simulink model "Monorail_Auxiliary_Power_Unit"  (R2021b)
settings: Solver=ode1  StartTime=0.0  StopTime=2.00  FixedStep=1e-06  MaxStep=1e-4  RelTol=1e-3
InitFcn:
  | %Input
  | V_supply_max = 910;
  | V_supply_min = 490;
  | V_supply_nom = 750;
  | R_supply = 1e-06;
  | L_in = 0.5e-03;
  | C_in = 215e-06;
  | R_Precharge = 1;
  | 
  | %PSFB_Voltage_Control
  | t_psfb_on = 0.05;
  | f_sw = 10e03;
  | V_dc_ref = 700;
  | V_dc_init = 450;
  | V_bat_ref = 24;
  | V_bat_init = 14;
  | Count_prd = 5000;
  | Half_prd = 2500;
  | Half_prd_fix = 2700;
  | Half_prd_var = 2300;
  | t_softstart = 100e-03;
  | Scale_factor_High = 1/737;
  | Scale_factor_Low = 1/48;
  | Kp_psfb = 2;
  | Ki_psfb =20;
  | Kp_feed = 0.00001;
  | PI_max = 1;
  | PI_min = 0;
  | t_enable = 1e-03;
  | Dead_prd = 1e-03
  | 
  | %PSFB_Current_Control
  | Scale_factor_i = 1/800;
  | I_cnst = 450;
  | I_over = 460;
  | Kp_psfb_i = 10;
  | Ki_psfb_i = 20;
  | 
  | %HF_Transformer
  | P_txf = 50e03;
  | f_txf = 10e03;
  | V_pri_txf = 1e03;
  | V_sec_high_txf = 720;
  | V_sec_low_txf = 27;
  | 
  | %DC_Link
  | L_filt = 1e-03;
  | C_filt = 215e-06;
  | R_Bleeder_700V = 0.5e03;
  | R_Bleeder_24V = 1e03
  | 
  | %Inverter_Control
  | t_inv_on = 1.5;
  | f_fund = 50;
  | V_phase_ref = 240;
  | Scale_factor_inv = 1/50e03;
  | Kp_inv = 0.05;
  | Ki_inv = 0.1;
  | PI_inv_max = 1;
  | PI_inv_min = -1;
  | ... (+27 lines)
undefined symbols (not defined in the file): Ion, Lithium
libraries: spsSeriesRLCBranchLib x35, spsIGBTDiodeLib x14, spsDiodeLib x13, spsMeanLib x11, spsBreakerLib x9, spsVoltageMeasurementLib x9, simulink x8, spsRMSLib x8, spsCurrentMeasurementLib x6, dspfdesign x6, spsabctodq0Lib x4, spsLinearTransformerLib x2
(part 2 of 3)

== system Monorail_Auxiliary_Power_Unit/First Stage/PSFB Pulse Generator/Loop Select ==
  Fixed Pulses Voltage Loop : Inport
  Variable Pulses Volatge Loop : Inport  Port=2
  OverCurrent Status : Inport  Port=3
  Fixed Pulses Current Loop : Inport  Port=4
  Variable Pulses Current Loop : Inport  Port=5
  Switch : Switch  Criteria=u2 > Threshold
  Switch1 : Switch  Criteria=u2 > Threshold
  Fixed Pulses : Outport
  Variable Pulses : Outport  Port=2
  wires:
  Switch/1 -> Fixed Pulses/1
  OverCurrent Status/1 -> Switch/2, Switch1/2
  Variable Pulses Current Loop/1 -> Switch1/3
  Variable Pulses Volatge Loop/1 -> Switch1/1
  Fixed Pulses Voltage Loop/1 -> Switch/1
  Switch1/1 -> Variable Pulses/1
  Fixed Pulses Current Loop/1 -> Switch/3

== system Monorail_Auxiliary_Power_Unit/First Stage/PSFB Pulse Generator/Voltage Loop ==
  Vi : Inport
  Vo 700V : Inport  Port=2
  Vo 24V : Inport  Port=3
  Fbk Sel : Inport  Port=4
  Carrier Wave Generator : Subsystem
  Close Loop : Subsystem
  Comparator : Subsystem
  Modulating Wave Generator : Subsystem
  Pulses for Fixed PSFB : Subsystem
  Pulses for Variable PSFB : Subsystem
  Fixed Pulses : Outport
  Variable Pulses : Outport  Port=2
  wires:
  Pulses for Fixed PSFB/1(Fixed Pulses) -> Fixed Pulses/1
  Comparator/1(Fixed PSFB R Top Pulse) -> Pulses for Fixed PSFB/1(Fixed PSFB R Top Pulse)
  Carrier Wave Generator/1(Carrier Wave) -> Comparator/1(Carrier Wave)
  Fbk Sel/1 -> Close Loop/4(Fbk Sel)
  Close Loop/1(Phase Shift) -> Pulses for Variable PSFB/2(Phase Shift)
  Modulating Wave Generator/2(Variable Modulating Wave) -> Comparator/3(Variable Modulating Wave)
  Vo 24V/1 -> Close Loop/3(Vdc 24V)
  Modulating Wave Generator/1(Fixed Modulating Wave) -> Comparator/2(Fixed Modulating Wave)
  Vo 700V/1 -> Close Loop/2(Vdc 700V)
  Comparator/2(Variable PSFB R Top Pulse) -> Pulses for Variable PSFB/1(Variable PSFB R Top Pulse)
  Pulses for Variable PSFB/1(Variable Pulses) -> Variable Pulses/1
  Vi/1 -> Close Loop/1(Vi)

== system Monorail_Auxiliary_Power_Unit/Second Stage/Pulse Generator/Current Loop ==
  I fbk : Inport
  I Feedback : Subsystem
  I Modulation Index : Display
  I PI Block : Subsystem
  I Reference : Subsystem
  Overcurrent Status Check : Subsystem
  I PI Out : Outport
  I Theta : Outport  Port=2
  Inverter Overcurrent Status : Outport  Port=3
  wires:
  I PI Block/1(I PI Out) -> I PI Out/1
  I Feedback/1(I dq0) -> I PI Block/2(I Feedback)
  I fbk/1 -> I Feedback/1(I fbk), Overcurrent Status Check/1(I fbk)
  I Reference/2(I ThetaIdeal) -> [ITheta]
  [ITheta] -> I Feedback/2(I Theta), I Theta/1
  I Reference/1(I dq0) -> I PI Block/1(I Reference)
  I PI Block/2(I Modulation Index) -> I Modulation Index/1
  Overcurrent Status Check/1(Inverter Overcurrent Status) -> Inverter Overcurrent Status/1

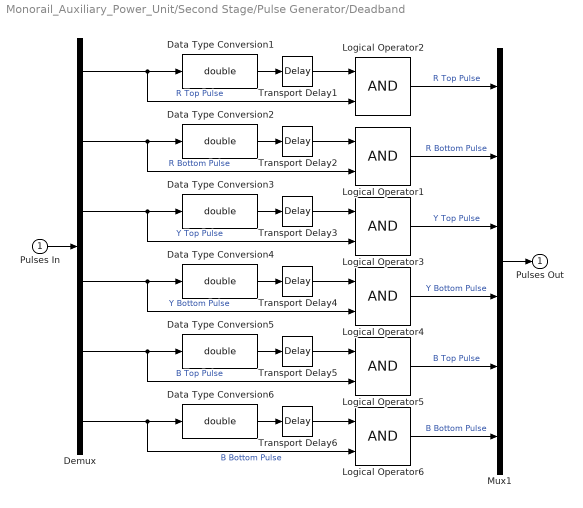
== system Monorail_Auxiliary_Power_Unit/Second Stage/Pulse Generator/Deadband ==
  Pulses In : Inport
  Data Type Conversion{1..6} (6 alike) : DataTypeConversion  OutDataTypeStr=double
  Demux : Demux  Outputs=6
  Logical Operator{1..6} (6 alike) : Logic  IconShape=distinctive  AllPortsSameDT=off  OutDataTypeStr=boolean
  Mux1 : Mux  Inputs=6
  Transport Delay{1..6} (6 alike) : TransportDelay  DelayTime=t_dead
  Pulses Out : Outport
  wires:
  Transport Delay2/1 -> Logical Operator1/1
  Data Type Conversion4/1 -> Transport Delay4/1
  Transport Delay3/1 -> Logical Operator3/1
  Transport Delay5/1 -> Logical Operator5/1
  Demux/2 -> Logical Operator1/2, Data Type Conversion2/1  "R Bottom Pulse"
  Data Type Conversion1/1 -> Transport Delay1/1
  Demux/1 -> Logical Operator2/2, Data Type Conversion1/1  "R Top Pulse"
  Transport Delay1/1 -> Logical Operator2/1
  Demux/4 -> Logical Operator4/2, Data Type Conversion4/1  "Y Bottom Pulse"
  Data Type Conversion3/1 -> Transport Delay3/1
  Transport Delay4/1 -> Logical Operator4/1
  Demux/3 -> Logical Operator3/2, Data Type Conversion3/1  "Y Top Pulse"
  Data Type Conversion2/1 -> Transport Delay2/1
  Data Type Conversion5/1 -> Transport Delay5/1
  Demux/5 -> Logical Operator5/2, Data Type Conversion5/1  "B Top Pulse"
  Demux/6 -> Logical Operator6/2, Data Type Conversion6/1  "B Bottom Pulse"
  Transport Delay6/1 -> Logical Operator6/1
  Data Type Conversion6/1 -> Transport Delay6/1
  Mux1/1 -> Pulses Out/1
  Logical Operator3/1 -> Mux1/3  "Y Top Pulse"
  Logical Operator2/1 -> Mux1/1  "R Top Pulse"
  Logical Operator5/1 -> Mux1/5  "B Top Pulse"
  Logical Operator1/1 -> Mux1/2  "R Bottom Pulse"
  Logical Operator4/1 -> Mux1/4  "Y Bottom Pulse"
  Logical Operator6/1 -> Mux1/6  "B Bottom Pulse"
  Pulses In/1 -> Demux/1

== system Monorail_Auxiliary_Power_Unit/Second Stage/Pulse Generator/Loop Select ==
  I PI : Inport
  I Theta : Inport  Port=2
  Inverter Overcurrent Status : Inport  Port=3
  V PI : Inport  Port=4
  V Theta : Inport  Port=5
  DQ0 Switch : Switch  Criteria=u2 > Threshold  Threshold=1/2
  Theta Switch : Switch  Criteria=u2 > Threshold  Threshold=1/2
  DQ0 : Outport
  Theta : Outport  Port=2
  wires:
  V Theta/1 -> Theta Switch/3
  Inverter Overcurrent Status/1 -> DQ0 Switch/2, Theta Switch/2
  I PI/1 -> DQ0 Switch/1
  V PI/1 -> DQ0 Switch/3
  DQ0 Switch/1 -> DQ0/1
  Theta Switch/1 -> Theta/1
  I Theta/1 -> Theta Switch/1

== system Monorail_Auxiliary_Power_Unit/Second Stage/Pulse Generator/Pulse ==
  dq0 : Inport
  Theta : Inport  Port=2
  Gate Pulses : Subsystem
  IPARK_MACRO : Subsystem
  SVGEN_DQ : Subsystem
  Pulses : Outport
  wires:
  SVGEN_DQ/1(SW) -> Gate Pulses/1(SW)
  Gate Pulses/1(Pulses) -> Pulses/1
  IPARK_MACRO/1(Alpha) -> SVGEN_DQ/1(Alpha)
  IPARK_MACRO/2(Beta) -> SVGEN_DQ/2(Beta)
  dq0/1 -> IPARK_MACRO/1(DQ0)
  Theta/1 -> IPARK_MACRO/2(Theta)

== system Monorail_Auxiliary_Power_Unit/Second Stage/Pulse Generator/Voltage Loop ==
  V fbk : Inport
  V Feedback : Subsystem
  V Modulation Index : Display
  V PI Block : Subsystem
  V Reference : Subsystem
  V PI Out : Outport
  V Theta : Outport  Port=2
  wires:
  V PI Block/2(V Modulation Index) -> V Modulation Index/1
  V Reference/1(V dq0) -> V PI Block/1(V Reference)
  [VTheta] -> V Theta/1, V Feedback/2(Theta)
  V Reference/2(V ThetaIdeal) -> [VTheta]
  V fbk/1 -> V Feedback/1(fbk)
  V Feedback/1(dq0) -> V PI Block/2(V Feedback)
  V PI Block/1(V PI Out) -> V PI Out/1

== system Monorail_Auxiliary_Power_Unit/First Stage/PSFB Pulse Generator/Current Loop/Carrier Wave Generator ==
  Repeating Sequence : simulink/Sources/Repeating Sequence  rep_seq_t=[0 (1/f_sw)/2 1/f_sw]  rep_seq_y=[0 Count_prd 0]
  Saturation5 : Saturate  UpperLimit=Count_prd  LowerLimit=0
  Carrier Wave : Outport
  wires:
  Saturation5/1 -> Carrier Wave/1  "Limited Carrier Wave"
  Repeating Sequence/1 -> Saturation5/1  "Carrier Wave"

== system Monorail_Auxiliary_Power_Unit/First Stage/PSFB Pulse Generator/Current Loop/Close Loop ==
  Ibat : Inport
  Error Signal Generator : Subsystem
  OverCurrent Fault Check : Subsystem
  PI Controller : Subsystem
  Duty : Outport
  OverCurrent Status : Outport  Port=2
  wires:
  Ibat/1 -> OverCurrent Fault Check/1(I bat), Error Signal Generator/1(Ibat)
  OverCurrent Fault Check/1(OverCurrent Status) -> OverCurrent Status/1
  PI Controller/1(Duty) -> Duty/1
  Error Signal Generator/1(Error Signal) -> PI Controller/1(Error Signal)

== system Monorail_Auxiliary_Power_Unit/First Stage/PSFB Pulse Generator/Current Loop/Comparator ==
  Carrier Wave : Inport
  Fixed Modulating Wave : Inport  Port=2
  Variable Modulating Wave : Inport  Port=3
  Relational Operator2 : RelationalOperator  OutDataTypeStr=boolean  RndMeth=Nearest
  Relational Operator3 : RelationalOperator  Operator=<=  OutDataTypeStr=boolean  RndMeth=Nearest
  Fixed PSFB R Top Pulse : Outport
  Variable PSFB R Top Pulse : Outport  Port=2
  wires:
  Variable Modulating Wave/1 -> Relational Operator3/2
  Relational Operator3/1 -> Variable PSFB R Top Pulse/1  "Pulse"
  Relational Operator2/1 -> Fixed PSFB R Top Pulse/1  "Pulse"
  Carrier Wave/1 -> Relational Operator2/1, Relational Operator3/1
  Fixed Modulating Wave/1 -> Relational Operator2/2

== system Monorail_Auxiliary_Power_Unit/First Stage/PSFB Pulse Generator/Current Loop/Modulating Wave Generator ==
  Duty : Inport
  Constant2 : Constant  Value=Half_prd_fix
  Constant3 : Constant  Value=Half_prd_var
  Saturation : Saturate  UpperLimit=Half_prd_var  LowerLimit=0
  Saturation1 : Saturate  UpperLimit=Count_prd  LowerLimit=Half_prd_fix
  Sum3 : Sum  Inputs=|+-
  Sum4 : Sum  Inputs=|++
  Fixed Modulating Wave : Outport
  Variable Modulating Wave : Outport  Port=2
  wires:
  Duty/1 -> Sum4/2, Sum3/2
  Constant2/1 -> Sum4/1
  Constant3/1 -> Sum3/1
  Sum4/1 -> Saturation1/1
  Sum3/1 -> Saturation/1
  Saturation/1 -> Variable Modulating Wave/1
  Saturation1/1 -> Fixed Modulating Wave/1

== system Monorail_Auxiliary_Power_Unit/First Stage/PSFB Pulse Generator/Current Loop/Pulses for Fixed PSFB ==
  Fixed PSFB R Top Pulse : Inport
  Data Type Conversion1 : DataTypeConversion  OutDataTypeStr=boolean
  Data Type Conversion6 : DataTypeConversion  OutDataTypeStr=double
  Mux : Mux  Inputs=2
  Rate Transition : RateTransition  Commented=through
  Transport Delay1 : TransportDelay  DelayTime=(180/360)*(1/f_sw)
  Fixed Pulses : Outport
  wires:
  Fixed PSFB R Top Pulse/1 -> Mux/1, Data Type Conversion6/1  "Fixed PSFB R Top Pulse"
  Data Type Conversion1/1 -> Mux/2  "Fixed PSFB Y Top Pulse"
  Rate Transition/1 -> Fixed Pulses/1
  Mux/1 -> Rate Transition/1
  Transport Delay1/1 -> Data Type Conversion1/1
  Data Type Conversion6/1 -> Transport Delay1/1

== system Monorail_Auxiliary_Power_Unit/First Stage/PSFB Pulse Generator/Current Loop/Pulses for Variable PSFB ==
  Fixed PSFB R Top Pulse : Inport
  Data Type Conversion1 : DataTypeConversion  OutDataTypeStr=boolean
  Data Type Conversion6 : DataTypeConversion  OutDataTypeStr=double
  Mux : Mux  Inputs=2
  Rate Transition : RateTransition  Commented=through
  Transport Delay1 : TransportDelay  DelayTime=(180/360)*(1/f_sw)
  Fixed Pulses : Outport
  wires:
  Data Type Conversion6/1 -> Transport Delay1/1
  Transport Delay1/1 -> Data Type Conversion1/1
  Mux/1 -> Rate Transition/1
  Rate Transition/1 -> Fixed Pulses/1
  Data Type Conversion1/1 -> Mux/2  "Fixed PSFB Y Top Pulse"
  Fixed PSFB R Top Pulse/1 -> Data Type Conversion6/1, Mux/1  "Fixed PSFB R Top Pulse"

== system Monorail_Auxiliary_Power_Unit/First Stage/PSFB Pulse Generator/Voltage Loop/Carrier Wave Generator ==
  Repeating Sequence : simulink/Sources/Repeating Sequence  rep_seq_t=[0 (1/f_sw)/2 1/f_sw]  rep_seq_y=[0 Count_prd 0]
  Saturation5 : Saturate  UpperLimit=Count_prd  LowerLimit=0
  Carrier Wave : Outport
  wires:
  Repeating Sequence/1 -> Saturation5/1  "Carrier Wave"
  Saturation5/1 -> Carrier Wave/1  "Limited Carrier Wave"

== system Monorail_Auxiliary_Power_Unit/First Stage/PSFB Pulse Generator/Voltage Loop/Close Loop ==
  Vi : Inport
  Vdc 700V : Inport  Port=2
  Vdc 24V : Inport  Port=3
  Fbk Sel : Inport  Port=4
  Feedback : Subsystem
  Feedforward : Subsystem
  Gain6 : Gain  Gain=(180/360)*(1/f_sw)
  Sum : Sum  Inputs=|++
  Phase Shift : Outport
  wires:
  Vdc 700V/1 -> Feedback/1(Vdc 700V)
  Vdc 24V/1 -> Feedback/2(Vdc 24V)
  Fbk Sel/1 -> Feedback/3(Fbk Sel)
  Feedback/1(PI Out) -> Sum/2
  Sum/1 -> Gain6/1
  Gain6/1 -> Phase Shift/1
  Vi/1 -> Feedforward/1(V supply)
  Feedforward/1(P Out) -> Sum/1

== system Monorail_Auxiliary_Power_Unit/First Stage/PSFB Pulse Generator/Voltage Loop/Comparator ==
  Carrier Wave : Inport
  Fixed Modulating Wave : Inport  Port=2
  Variable Modulating Wave : Inport  Port=3
  Relational Operator2 : RelationalOperator  OutDataTypeStr=boolean  RndMeth=Nearest
  Relational Operator3 : RelationalOperator  Operator=<=  OutDataTypeStr=boolean  RndMeth=Nearest
  Fixed PSFB R Top Pulse : Outport
  Variable PSFB R Top Pulse : Outport  Port=2
  wires:
  Fixed Modulating Wave/1 -> Relational Operator2/2
  Carrier Wave/1 -> Relational Operator3/1, Relational Operator2/1
  Relational Operator2/1 -> Fixed PSFB R Top Pulse/1  "Pulse"
  Relational Operator3/1 -> Variable PSFB R Top Pulse/1  "Pulse"
  Variable Modulating Wave/1 -> Relational Operator3/2

== system Monorail_Auxiliary_Power_Unit/First Stage/PSFB Pulse Generator/Voltage Loop/Modulating Wave Generator ==
  Constant1 : Constant  Value=Count_prd
  Ramp2 : simulink/Sources/Ramp  slope=((Count_prd/2)-Dead_prd)/t_softstart  start=0  InitialOutput=0
  Saturation : Saturate  UpperLimit=Half_prd_var  LowerLimit=0
  Saturation4 : Saturate  UpperLimit=Count_prd  LowerLimit=Half_prd_fix
  Saturation6 : Saturate  UpperLimit=Half_prd_var  LowerLimit=0
  Sum2 : Sum  Inputs=|+-
  Fixed Modulating Wave : Outport
  Variable Modulating Wave : Outport  Port=2
  wires:
  Saturation/1 -> Sum2/2, Saturation6/1  "Actual Modulating Wave"
  Sum2/1 -> Saturation4/1  "Actual Modulating Wave"
  Saturation4/1 -> Fixed Modulating Wave/1  "Saturated Modulating Wave"
  Constant1/1 -> Sum2/1  "TBPRD"
  Ramp2/1 -> Saturation/1  "Initial Modulating Wave"
  Saturation6/1 -> Variable Modulating Wave/1  "Saturated Modulating Wave"

== system Monorail_Auxiliary_Power_Unit/First Stage/PSFB Pulse Generator/Voltage Loop/Pulses for Fixed PSFB ==
  Fixed PSFB R Top Pulse : Inport
  Data Type Conversion1 : DataTypeConversion  OutDataTypeStr=boolean
  Data Type Conversion6 : DataTypeConversion  OutDataTypeStr=double
  Mux : Mux  Inputs=2
  Rate Transition : RateTransition
  Transport Delay1 : TransportDelay  DelayTime=(180/360)*(1/f_sw)
  Fixed Pulses : Outport
  wires:
  Data Type Conversion6/1 -> Transport Delay1/1
  Transport Delay1/1 -> Data Type Conversion1/1
  Mux/1 -> Rate Transition/1
  Rate Transition/1 -> Fixed Pulses/1
  Data Type Conversion1/1 -> Mux/2  "Fixed PSFB Y Top Pulse"
  Fixed PSFB R Top Pulse/1 -> Data Type Conversion6/1, Mux/1  "Fixed PSFB R Top Pulse"

== system Monorail_Auxiliary_Power_Unit/First Stage/PSFB Pulse Generator/Voltage Loop/Pulses for Variable PSFB ==
  Variable PSFB R Top Pulse : Inport
  Phase Shift : Inport  Port=2
  Data Type Conversion2 : DataTypeConversion  OutDataTypeStr=double
  Data Type Conversion3 : DataTypeConversion  OutDataTypeStr=boolean
  Data Type Conversion5 : DataTypeConversion  OutDataTypeStr=boolean
  Mux1 : Mux  Inputs=2
  Rate Transition1 : RateTransition
  Transport Delay2 : TransportDelay  DelayTime=(180/360)*(1/f_sw)
  Variable Transport Delay : VariableTransportDelay  MaximumDelay=1/f_sw
  Variable Pulses : Outport
  wires:
  Phase Shift/1 -> Variable Transport Delay/2
  Data Type Conversion5/1 -> Mux1/1  "Variable PSFB R Top Pulse"
  Mux1/1 -> Rate Transition1/1
  Transport Delay2/1 -> Data Type Conversion3/1
  Variable PSFB R Top Pulse/1 -> Data Type Conversion2/1
  Data Type Conversion3/1 -> Mux1/2  "Variable PSFB Y Top Pulse"
  Data Type Conversion2/1 -> Variable Transport Delay/1
  Variable Transport Delay/1 -> Data Type Conversion5/1, Transport Delay2/1
  Rate Transition1/1 -> Variable Pulses/1

== system Monorail_Auxiliary_Power_Unit/Second Stage/Pulse Generator/Current Loop/I Feedback ==
  I fbk : Inport
  I Theta : Inport  Port=2
  Demux : Demux  Outputs=3
  Gain5 : Gain  Gain=Scale_factor_Iinv
  Lowpass Filter BR : dspfdesign/Lowpass Filter  Commented=through  FilterType=FIR  DesignForMinimumOrder=on  FilterOrder=50  PassbandFrequency=50  StopbandFrequency=1e03  PassbandRipple=0.1  StopbandAttenuation=100  InheritSampleRate=off  SampleRate=44100  SimulateUsing=Interpreted execution  roundingMode=Floor  coeffsDataTypeStr=fixdt(1,16)
  Lowpass Filter RY : dspfdesign/Lowpass Filter  Commented=through  FilterType=FIR  DesignForMinimumOrder=on  FilterOrder=50  PassbandFrequency=50  StopbandFrequency=1e03  PassbandRipple=0.1  StopbandAttenuation=100  InheritSampleRate=off  SampleRate=44100  SimulateUsing=Interpreted execution  roundingMode=Floor  coeffsDataTypeStr=fixdt(1,16)
  Lowpass Filter YB : dspfdesign/Lowpass Filter  Commented=through  FilterType=FIR  DesignForMinimumOrder=on  FilterOrder=50  PassbandFrequency=50  StopbandFrequency=1e03  PassbandRipple=0.1  StopbandAttenuation=100  InheritSampleRate=off  SampleRate=44100  SimulateUsing=Interpreted execution  roundingMode=Floor  coeffsDataTypeStr=fixdt(1,16)
  Mux : Mux  Inputs=3
  abc to dq0 : spsabctodq0Lib/abc to dq0  Alignment=90 degrees behind phase A axis
  I dq0 : Outport
  wires:
  I fbk/1 -> Demux/1
  Demux/3 -> Lowpass Filter BR/1
  Demux/2 -> Lowpass Filter YB/1
  Demux/1 -> Lowpass Filter RY/1
  Lowpass Filter BR/1 -> Mux/3
  Lowpass Filter YB/1 -> Mux/2
  Lowpass Filter RY/1 -> Mux/1
  I Theta/1 -> abc to dq0/2
  Mux/1 -> Gain5/1
  abc to dq0/1 -> I dq0/1
  Gain5/1 -> abc to dq0/1

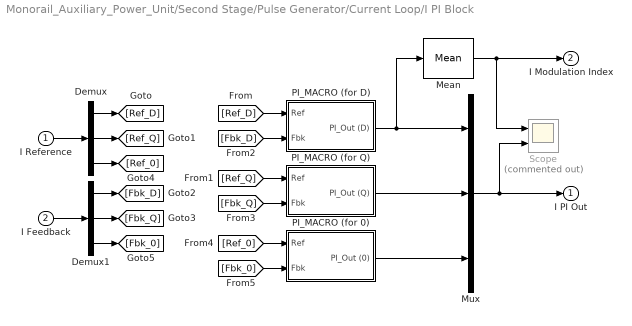
== system Monorail_Auxiliary_Power_Unit/Second Stage/Pulse Generator/Current Loop/I PI Block ==
  I Reference : Inport
  I Feedback : Inport  Port=2
  Demux : Demux  Outputs=3
  Demux1 : Demux  Outputs=3
  Mean : spsMeanLib/Mean  Freq=f_fund  Vinit=0  Ts=0
  Mux : Mux  Inputs=3
  PI_MACRO (for 0) : Subsystem
  PI_MACRO (for D) : Subsystem
  PI_MACRO (for Q) : Subsystem
  Scope : Scope  Commented=on  NumInputPorts=2
  I PI Out : Outport
  I Modulation Index : Outport  Port=2
  wires:
  PI_MACRO (for D)/1(PI_Out (D)) -> Mux/1, Mean/1
  Mean/1 -> I Modulation Index/1, Scope/1
  PI_MACRO (for 0)/1(PI_Out (0)) -> Mux/3
  [Ref_0] -> PI_MACRO (for 0)/1(Ref)
  [Fbk_0] -> PI_MACRO (for 0)/2(Fbk)
  I Reference/1 -> Demux/1
  I Feedback/1 -> Demux1/1
  [Fbk_Q] -> PI_MACRO (for Q)/2(Fbk)
  Demux1/2 -> [Fbk_Q]
  [Fbk_D] -> PI_MACRO (for D)/2(Fbk)
  Demux1/1 -> [Fbk_D]
  [Ref_Q] -> PI_MACRO (for Q)/1(Ref)
  Demux/2 -> [Ref_Q]
  [Ref_D] -> PI_MACRO (for D)/1(Ref)
  Demux/1 -> [Ref_D]
  Demux/3 -> [Ref_0]
  Demux1/3 -> [Fbk_0]
  PI_MACRO (for Q)/1(PI_Out (Q)) -> Mux/2
  Mux/1 -> Scope/2, I PI Out/1

== system Monorail_Auxiliary_Power_Unit/Second Stage/Pulse Generator/Current Loop/I Reference ==
  Constant : Constant  Value=2*pi/3
  Gain1 : Gain  Gain=I_Line_ref*sqrt(2)
  Gain2 : Gain  Gain=Scale_factor_Iinv
  Gain3 : Gain  Gain=I_Line_ref*sqrt(2)
  Gain4 : Gain  Gain=I_Line_ref*sqrt(2)
  I Theta : simulink/Sources/Repeating Sequence  rep_seq_t=[0 1/f_fund]  rep_seq_y=[0 2*pi]
  Mux2 : Mux  Inputs=3
  Sum1 : Sum  Inputs=|+-
  Sum2 : Sum  Inputs=|++
  Trigonometric Function : Trigonometry
  Trigonometric Function1 : Trigonometry
  Trigonometric Function2 : Trigonometry
  abc to dq0 : spsabctodq0Lib/abc to dq0  Alignment=90 degrees behind phase A axis
  I dq0 : Outport
  I ThetaIdeal : Outport  Port=2
  wires:
  [IThetaIdeal] -> I ThetaIdeal/1, abc to dq0/2
  Gain3/1 -> Mux2/2
  Gain1/1 -> Mux2/1
  Gain4/1 -> Mux2/3
  Gain2/1 -> abc to dq0/1
  I Theta/1 -> Sum2/1, Sum1/1, [IThetaIdeal], Trigonometric Function/1
  Mux2/1 -> Gain2/1
  abc to dq0/1 -> I dq0/1
  Constant/1 -> Sum1/2, Sum2/2
  Sum2/1 -> Trigonometric Function2/1
  Trigonometric Function/1 -> Gain1/1  "R"
  Trigonometric Function1/1 -> Gain3/1  "Y"
  Trigonometric Function2/1 -> Gain4/1  "B"
  Sum1/1 -> Trigonometric Function1/1

== system Monorail_Auxiliary_Power_Unit/Second Stage/Pulse Generator/Current Loop/Overcurrent Status Check ==
  I fbk : Inport
  Constant : Constant  Value=Iinvov
  Demux : Demux  Outputs=3
  GreaterThan1 : RelationalOperator  Operator=>  OutDataTypeStr=boolean  RndMeth=Simplest
  GreaterThan2 : RelationalOperator  Operator=>  OutDataTypeStr=boolean  RndMeth=Simplest
  GreaterThan3 : RelationalOperator  Operator=>  OutDataTypeStr=boolean  RndMeth=Simplest
  Logical Operator : Logic  Operator=OR  Inputs=3  IconShape=distinctive  AllPortsSameDT=off  OutDataTypeStr=boolean
  RMS1 : spsRMSLib/RMS  TrueRMS=on  Freq=f_fund  RMSInit=0  Ts=0
  RMS2 : spsRMSLib/RMS  TrueRMS=on  Freq=f_fund  RMSInit=0  Ts=0
  RMS3 : spsRMSLib/RMS  TrueRMS=on  Freq=f_fund  RMSInit=0  Ts=0
  Inverter Overcurrent Status : Outport
  wires:
  RMS1/1 -> GreaterThan1/1
  RMS2/1 -> GreaterThan2/1
  RMS3/1 -> GreaterThan3/1
  Constant/1 -> GreaterThan3/2, GreaterThan1/2, GreaterThan2/2
  GreaterThan1/1 -> Logical Operator/2
  Demux/1 -> RMS3/1
  GreaterThan2/1 -> Logical Operator/3
  Demux/2 -> RMS1/1
  Demux/3 -> RMS2/1
  GreaterThan3/1 -> Logical Operator/1
  Logical Operator/1 -> Inverter Overcurrent Status/1
  I fbk/1 -> Demux/1

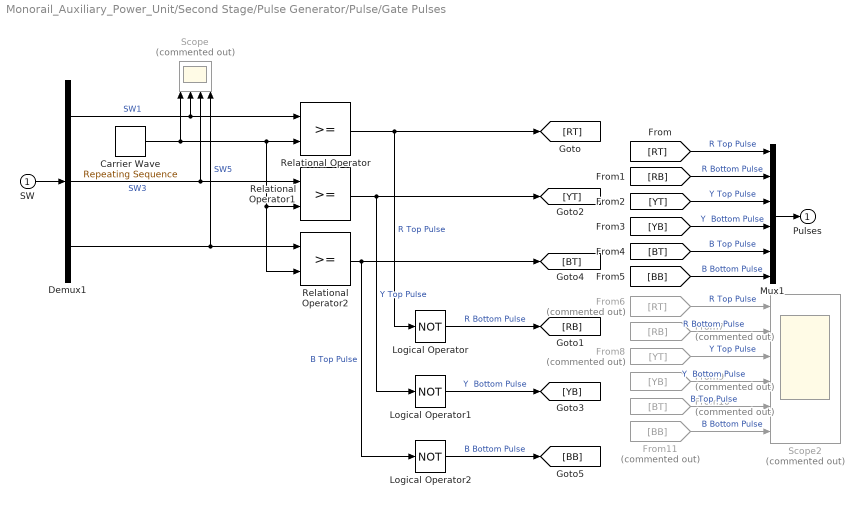
== system Monorail_Auxiliary_Power_Unit/Second Stage/Pulse Generator/Pulse/Gate Pulses ==
  SW : Inport
  Carrier Wave : simulink/Sources/Repeating Sequence  rep_seq_t=[0 (1/2e03)/2 1/2e03]  rep_seq_y=[0 1 0]
  Demux1 : Demux  Outputs=3
  From10 : From  Commented=on  GotoTag=BT
  From11 : From  Commented=on  GotoTag=BB
  From6 : From  Commented=on  GotoTag=RT
  From7 : From  Commented=on  GotoTag=RB
  From8 : From  Commented=on  GotoTag=YT
  From9 : From  Commented=on  GotoTag=YB
  Logical Operator : Logic  Operator=NOT  IconShape=distinctive  AllPortsSameDT=off  OutDataTypeStr=boolean
  Logical Operator1 : Logic  Operator=NOT  IconShape=distinctive  AllPortsSameDT=off  OutDataTypeStr=boolean
  Logical Operator2 : Logic  Operator=NOT  IconShape=distinctive  AllPortsSameDT=off  OutDataTypeStr=boolean
  Mux1 : Mux  Inputs=6
  Relational Operator : RelationalOperator  OutDataTypeStr=boolean  RndMeth=Nearest
  Relational Operator1 : RelationalOperator  OutDataTypeStr=boolean  RndMeth=Nearest
  Relational Operator2 : RelationalOperator  OutDataTypeStr=boolean  RndMeth=Nearest
  Scope : Scope  Commented=on  NumInputPorts=4
  Scope2 : Scope  Commented=on  NumInputPorts=6
  Pulses : Outport
  wires:
  Logical Operator/1 -> [RB]  "R Bottom Pulse"
  Logical Operator1/1 -> [YB]  "Y  Bottom Pulse"
  Demux1/2 -> Scope/3, Relational Operator1/1  "SW3"
  Demux1/3 -> Scope/4, Relational Operator2/1  "SW5"
  Logical Operator2/1 -> [BB]  "B Bottom Pulse"
  Demux1/1 -> Scope/2, Relational Operator/1  "SW1"
  Relational Operator2/1 -> [BT], Logical Operator2/1  "B Top Pulse"
  Relational Operator/1 -> Logical Operator/1, [RT]  "R Top Pulse"
  Carrier Wave/1 -> Relational Operator2/2, Relational Operator1/2, Relational Operator/2, Scope/1
  Relational Operator1/1 -> [YT], Logical Operator1/1  "Y Top Pulse"
  SW/1 -> Demux1/1
  Mux1/1 -> Pulses/1
  [YT] -> Mux1/3  "Y Top Pulse"
  [RT] -> Mux1/1  "R Top Pulse"
  [BT] -> Mux1/5  "B Top Pulse"
  [RB] -> Mux1/2  "R Bottom Pulse"
  [YB] -> Mux1/4  "Y  Bottom Pulse"
  [BB] -> Mux1/6  "B Bottom Pulse"
  From6/1 -> Scope2/1  "R Top Pulse"
  From7/1 -> Scope2/2  "R Bottom Pulse"
  From8/1 -> Scope2/3  "Y Top Pulse"
  From9/1 -> Scope2/4  "Y  Bottom Pulse"
  From10/1 -> Scope2/5  "B Top Pulse"
  From11/1 -> Scope2/6  "B Bottom Pulse"

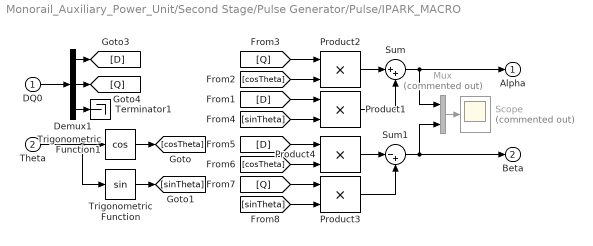
== system Monorail_Auxiliary_Power_Unit/Second Stage/Pulse Generator/Pulse/IPARK_MACRO ==
  DQ0 : Inport
  Theta : Inport  Port=2
  Demux1 : Demux  Outputs=3
  Mux : Mux  Commented=on  Inputs=2
  Product{1..4} (4 alike) : Product
  Scope : Scope  Commented=on
  Sum : Sum  Inputs=|++
  Sum1 : Sum  Inputs=|-+
  Terminator1 : Terminator
  Trigonometric Function : Trigonometry
  Trigonometric Function1 : Trigonometry  Operator=cos
  Alpha : Outport
  Beta : Outport  Port=2
  wires:
  Trigonometric Function1/1 -> [cosTheta]
  Trigonometric Function/1 -> [sinTheta]
  Theta/1 -> Trigonometric Function/1, Trigonometric Function1/1
  Demux1/3 -> Terminator1/1
  Demux1/1 -> [D]
  Demux1/2 -> [Q]
  Product2/1 -> Sum/1
  Product1/1 -> Sum/2
  Sum/1 -> Mux/1, Alpha/1
  Sum1/1 -> Beta/1, Mux/2
  Product3/1 -> Sum1/2
  Product4/1 -> Sum1/1
  [Q] -> Product2/1
  [cosTheta] -> Product2/2
  [D] -> Product1/1
  [sinTheta] -> Product1/2
  [D] -> Product4/1
  [cosTheta] -> Product4/2
  [Q] -> Product3/1
  [sinTheta] -> Product3/2
  DQ0/1 -> Demux1/1
  Mux/1 -> Scope/1

== system Monorail_Auxiliary_Power_Unit/Second Stage/Pulse Generator/Pulse/SVGEN_DQ ==
  Alpha : Inport
  Beta : Inport  Port=2
  Display : Display  Commented=on
  Scaling Block : Subsystem
  "Sector " : Scope  Commented=on
  Sector Determination : Subsystem
  Switching Time Calculation : Subsystem
  Temp calculation : Subsystem
  SW : Outport
  wires:
  Alpha/1 -> Temp calculation/1(Alpha)
  Sector Determination/1(Sector) -> Switching Time Calculation/2(Sector), "Sector "/1, Display/1
  Temp calculation/1(Temp) -> Switching Time Calculation/1(tmp), Sector Determination/1(Temp)
  Beta/1 -> Temp calculation/2(Beta)
  Switching Time Calculation/1(Switching Time) -> Scaling Block/1(In)
  Scaling Block/1(Out) -> SW/1

== system Monorail_Auxiliary_Power_Unit/Second Stage/Pulse Generator/Voltage Loop/V Feedback ==
  fbk : Inport
  Theta : Inport  Port=2
  Demux : Demux  Outputs=3
  Gain5 : Gain  Gain=Scale_factor_inv
  Lowpass Filter BR : dspfdesign/Lowpass Filter  Commented=through  FilterType=FIR  DesignForMinimumOrder=on  FilterOrder=50  PassbandFrequency=f_fund  StopbandFrequency=1e03  PassbandRipple=0.1  StopbandAttenuation=100  InheritSampleRate=off  SampleRate=44100  SimulateUsing=Interpreted execution  roundingMode=Floor  coeffsDataTypeStr=fixdt(1,16)
  Lowpass Filter RY : dspfdesign/Lowpass Filter  Commented=through  FilterType=FIR  DesignForMinimumOrder=on  FilterOrder=50  PassbandFrequency=f_fund  StopbandFrequency=1e03  PassbandRipple=0.1  StopbandAttenuation=100  InheritSampleRate=off  SampleRate=44100  SimulateUsing=Interpreted execution  roundingMode=Floor  coeffsDataTypeStr=fixdt(1,16)
  Lowpass Filter YB : dspfdesign/Lowpass Filter  Commented=through  FilterType=FIR  DesignForMinimumOrder=on  FilterOrder=50  PassbandFrequency=f_fund  StopbandFrequency=1e03  PassbandRipple=0.1  StopbandAttenuation=100  InheritSampleRate=off  SampleRate=44100  SimulateUsing=Interpreted execution  roundingMode=Floor  coeffsDataTypeStr=fixdt(1,16)
  Mux : Mux  Inputs=3
  abc to dq0 : spsabctodq0Lib/abc to dq0  Alignment=90 degrees behind phase A axis
  dq0 : Outport
  wires:
  Gain5/1 -> abc to dq0/1
  abc to dq0/1 -> dq0/1
  Mux/1 -> Gain5/1
  Theta/1 -> abc to dq0/2
  Lowpass Filter RY/1 -> Mux/1
  Lowpass Filter YB/1 -> Mux/2
  Lowpass Filter BR/1 -> Mux/3
  Demux/1 -> Lowpass Filter RY/1
  Demux/2 -> Lowpass Filter YB/1
  Demux/3 -> Lowpass Filter BR/1
  fbk/1 -> Demux/1

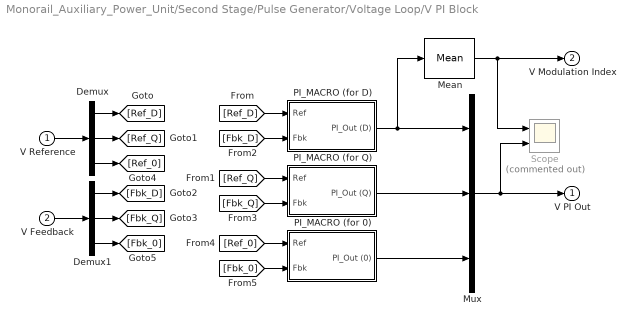
== system Monorail_Auxiliary_Power_Unit/Second Stage/Pulse Generator/Voltage Loop/V PI Block ==
  V Reference : Inport
  V Feedback : Inport  Port=2
  Demux : Demux  Outputs=3
  Demux1 : Demux  Outputs=3
  Mean : spsMeanLib/Mean  Freq=f_fund  Vinit=0  Ts=0
  Mux : Mux  Inputs=3
  PI_MACRO (for 0) : Subsystem
  PI_MACRO (for D) : Subsystem
  PI_MACRO (for Q) : Subsystem
  Scope : Scope  Commented=on  NumInputPorts=2
  V PI Out : Outport
  V Modulation Index : Outport  Port=2
  wires:
  Mux/1 -> V PI Out/1, Scope/2
  PI_MACRO (for Q)/1(PI_Out (Q)) -> Mux/2
  Demux1/3 -> [Fbk_0]
  Demux/3 -> [Ref_0]
  Demux/1 -> [Ref_D]
  [Ref_D] -> PI_MACRO (for D)/1(Ref)
  Demux/2 -> [Ref_Q]
  [Ref_Q] -> PI_MACRO (for Q)/1(Ref)
  Demux1/1 -> [Fbk_D]
  [Fbk_D] -> PI_MACRO (for D)/2(Fbk)
  Demux1/2 -> [Fbk_Q]
  [Fbk_Q] -> PI_MACRO (for Q)/2(Fbk)
  V Feedback/1 -> Demux1/1
  V Reference/1 -> Demux/1
  [Fbk_0] -> PI_MACRO (for 0)/2(Fbk)
  [Ref_0] -> PI_MACRO (for 0)/1(Ref)
  PI_MACRO (for 0)/1(PI_Out (0)) -> Mux/3
  Mean/1 -> Scope/1, V Modulation Index/1
  PI_MACRO (for D)/1(PI_Out (D)) -> Mean/1, Mux/1

== system Monorail_Auxiliary_Power_Unit/Second Stage/Pulse Generator/Voltage Loop/V Reference ==
  Constant : Constant  Value=2*pi/3
  Gain1 : Gain  Gain=V_phase_ref*sqrt(2)
  Gain2 : Gain  Gain=Scale_factor_inv
  Gain3 : Gain  Gain=V_phase_ref*sqrt(2)
  Gain4 : Gain  Gain=V_phase_ref*sqrt(2)
  Mux2 : Mux  Inputs=3
  Sum{,1,3..4} (4 alike) : Sum  Inputs=|+-
  Sum2 : Sum  Inputs=|++
  Trigonometric Function : Trigonometry
  Trigonometric Function1 : Trigonometry
  Trigonometric Function2 : Trigonometry
  V Theta : simulink/Sources/Repeating Sequence  rep_seq_t=[0 1/f_fund]  rep_seq_y=[0 2*pi]
  abc to dq0 : spsabctodq0Lib/abc to dq0  Alignment=90 degrees behind phase A axis
  V dq0 : Outport
  V ThetaIdeal : Outport  Port=2
  wires:
  Sum1/1 -> Trigonometric Function1/1
  Trigonometric Function2/1 -> Gain4/1  "B"
  Trigonometric Function1/1 -> Gain3/1  "Y"
  Trigonometric Function/1 -> Gain1/1  "R"
  Sum2/1 -> Trigonometric Function2/1
  Constant/1 -> Sum2/2, Sum1/2
  abc to dq0/1 -> V dq0/1
  Mux2/1 -> Gain2/1
  V Theta/1 -> Trigonometric Function/1, [VThetaIdeal], Sum1/1, Sum2/1
  Gain2/1 -> abc to dq0/1
  Sum4/1 -> Mux2/3
  Sum/1 -> Mux2/1
  Sum3/1 -> Mux2/2
  Gain1/1 -> Sum/1, Sum4/2
  Gain3/1 -> Sum/2, Sum3/1
  Gain4/1 -> Sum4/1, Sum3/2
  [VThetaIdeal] -> abc to dq0/2, V ThetaIdeal/1

== system Monorail_Auxiliary_Power_Unit/First Stage/PSFB Pulse Generator/Current Loop/Close Loop/Error Signal Generator ==
  Ibat : Inport
  Constant1 : Constant  Value=I_cnst
  Gain2 : Gain  Gain=Scale_factor_i
  Gain3 : Gain  Gain=Scale_factor_i
  Sum1 : Sum  Inputs=|+-
  Error Signal : Outport
  wires:
  Sum1/1 -> Error Signal/1
  Constant1/1 -> Gain2/1
  Gain3/1 -> Sum1/2
  Gain2/1 -> Sum1/1
  Ibat/1 -> Gain3/1

== system Monorail_Auxiliary_Power_Unit/First Stage/PSFB Pulse Generator/Current Loop/Close Loop/OverCurrent Fault Check ==
  I bat : Inport
  Constant : Constant  Value=I_over
  GreaterThan : RelationalOperator  Operator=>  OutDataTypeStr=boolean  RndMeth=Simplest
  OverCurrent Status : Outport
  wires:
  Constant/1 -> GreaterThan/2
  I bat/1 -> GreaterThan/1
  GreaterThan/1 -> OverCurrent Status/1

== system Monorail_Auxiliary_Power_Unit/First Stage/PSFB Pulse Generator/Current Loop/Close Loop/PI Controller ==
  Error Signal : Inport
  Gain : Gain  Gain=Ki_psfb_i
  Gain1 : Gain  Gain=Kp_psfb_i
  Integrator : Integrator
  Saturation2 : Saturate  UpperLimit=Half_prd  LowerLimit=0  ZeroCross=off
  Sum : Sum
  Sum2 : Sum  Inputs=|++
  Duty : Outport
  wires:
  Error Signal/1 -> Sum/1, Gain1/1
  Saturation2/1 -> Duty/1
  Sum/1 -> Gain/1, Integrator/1
  Sum2/1 -> Saturation2/1
  Integrator/1 -> Sum/2
  Gain1/1 -> Sum2/1
  Gain/1 -> Sum2/2

== system Monorail_Auxiliary_Power_Unit/First Stage/PSFB Pulse Generator/Voltage Loop/Close Loop/Feedback ==
  Vdc 700V : Inport
  Vdc 24V : Inport  Port=2
  Fbk Sel : Inport  Port=3
  Error Signal Generator : Subsystem
  PI Controller : Subsystem
  PI Out : Outport
  wires:
  Error Signal Generator/1(Error Signal) -> PI Controller/1(PI In)
  Vdc 700V/1 -> Error Signal Generator/1(V dc)
  Vdc 24V/1 -> Error Signal Generator/2(V bat)
  PI Controller/1(PI Out) -> PI Out/1
  Fbk Sel/1 -> Error Signal Generator/3(Fbk Sel)

== system Monorail_Auxiliary_Power_Unit/First Stage/PSFB Pulse Generator/Voltage Loop/Close Loop/Feedforward ==
  V supply : Inport
  Constant : Constant  Value=V_supply_nom
  Gain : Gain  Gain=Kp_feed
  Gain1 : Gain  Gain=Scale_factor_High
  Gain2 : Gain  Gain=Scale_factor_High
  Saturation2 : Saturate  UpperLimit=PI_max  LowerLimit=PI_min  ZeroCross=off
  Sum1 : Sum  Inputs=|+-
  P Out : Outport
  wires:
  Gain2/1 -> Sum1/1
  Constant/1 -> Gain2/1
  V supply/1 -> Gain1/1
  Gain1/1 -> Sum1/2
  Sum1/1 -> Gain/1
  Saturation2/1 -> P Out/1
  Gain/1 -> Saturation2/1

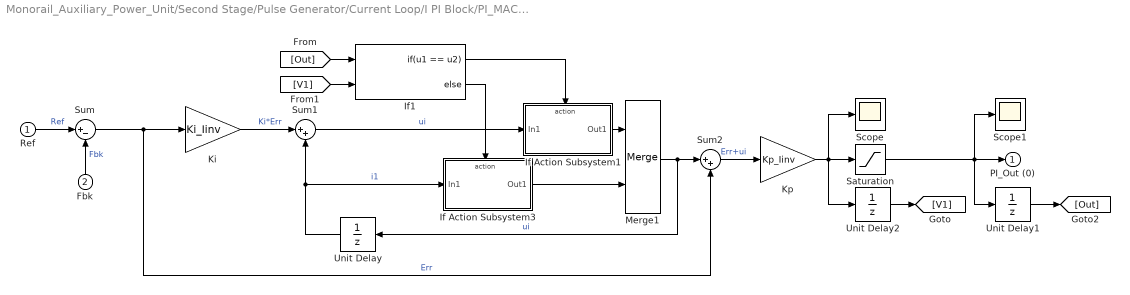
== system Monorail_Auxiliary_Power_Unit/Second Stage/Pulse Generator/Current Loop/I PI Block/PI_MACRO (for 0) ==
  Ref : Inport
  Fbk : Inport  Port=2
  If Action Subsystem1 : Subsystem  TreatAsAtomicUnit=on
  If Action Subsystem3 : Subsystem  TreatAsAtomicUnit=on
  If1 : If  NumInputs=2  IfExpression=u1 == u2
  Ki : Gain  Gain=Ki_Iinv
  Kp : Gain  Gain=Kp_Iinv
  Merge1 : Merge
  Saturation : Saturate  UpperLimit=PI_inv_max  LowerLimit=PI_inv_min
  Scope : Scope
  Scope1 : Scope
  Sum : Sum  Inputs=|+-
  Sum1 : Sum  Inputs=|++
  Sum2 : Sum  Inputs=|++
  Unit Delay : UnitDelay  SampleTime=-1  HasFrameUpgradeWarning=on
  Unit Delay1 : UnitDelay  SampleTime=-1  HasFrameUpgradeWarning=on
  Unit Delay2 : UnitDelay  SampleTime=-1  HasFrameUpgradeWarning=on
  PI_Out (0) : Outport
  wires:
  If Action Subsystem3/1(Out1) -> Merge1/2
  Sum2/1 -> Kp/1  "Err+ui"
  If1/2 -> If Action Subsystem3/Action
  Ref/1 -> Sum/1  "Ref"
  Ki/1 -> Sum1/1  "Ki*Err"
  Kp/1 -> Unit Delay2/1, Saturation/1, Scope/1
  [Out] -> If1/1
  If1/1 -> If Action Subsystem1/Action
  Unit Delay/1 -> If Action Subsystem3/1(In1), Sum1/2  "i1"
  [V1] -> If1/2
  Sum1/1 -> If Action Subsystem1/1(In1)  "ui"
  Fbk/1 -> Sum/2  "Fbk"
  Merge1/1 -> Sum2/1, Unit Delay/1  "ui"
  Sum/1 -> Ki/1, Sum2/2  "Err"
  If Action Subsystem1/1(Out1) -> Merge1/1
  Saturation/1 -> Unit Delay1/1, PI_Out (0)/1, Scope1/1
  Unit Delay1/1 -> [Out]
  Unit Delay2/1 -> [V1]

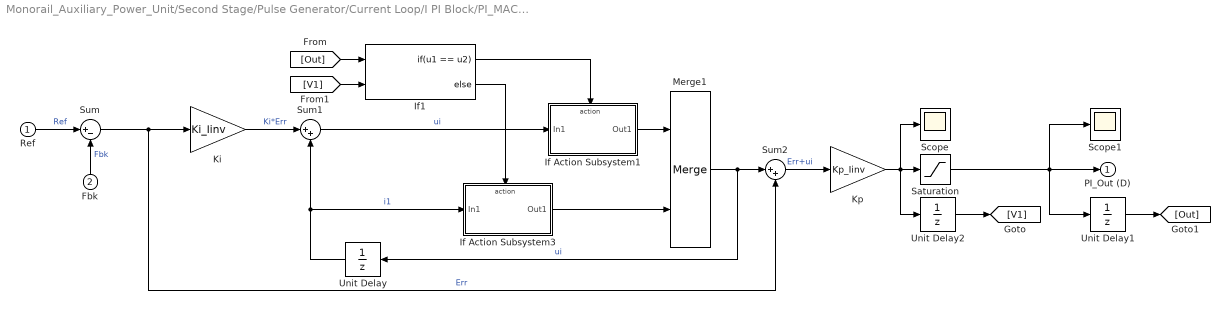
== system Monorail_Auxiliary_Power_Unit/Second Stage/Pulse Generator/Current Loop/I PI Block/PI_MACRO (for D) ==
  Ref : Inport
  Fbk : Inport  Port=2
  If Action Subsystem1 : Subsystem  TreatAsAtomicUnit=on
  If Action Subsystem3 : Subsystem  TreatAsAtomicUnit=on
  If1 : If  NumInputs=2  IfExpression=u1 == u2
  Ki : Gain  Gain=Ki_Iinv
  Kp : Gain  Gain=Kp_Iinv
  Merge1 : Merge
  Saturation : Saturate  UpperLimit=PI_inv_max  LowerLimit=PI_inv_min
  Scope : Scope
  Scope1 : Scope
  Sum : Sum  Inputs=|+-
  Sum1 : Sum  Inputs=|++
  Sum2 : Sum  Inputs=|++
  Unit Delay : UnitDelay  SampleTime=-1  HasFrameUpgradeWarning=on
  Unit Delay1 : UnitDelay  SampleTime=-1  HasFrameUpgradeWarning=on
  Unit Delay2 : UnitDelay  SampleTime=-1  HasFrameUpgradeWarning=on
  PI_Out (D) : Outport
  wires:
  Unit Delay2/1 -> [V1]
  Unit Delay1/1 -> [Out]
  If Action Subsystem3/1(Out1) -> Merge1/2
  Sum2/1 -> Kp/1  "Err+ui"
  If1/2 -> If Action Subsystem3/Action
  Ref/1 -> Sum/1  "Ref"
  Ki/1 -> Sum1/1  "Ki*Err"
  Kp/1 -> Unit Delay2/1, Scope/1, Saturation/1
  [Out] -> If1/1
  If1/1 -> If Action Subsystem1/Action
  Unit Delay/1 -> If Action Subsystem3/1(In1), Sum1/2  "i1"
  [V1] -> If1/2
  Sum1/1 -> If Action Subsystem1/1(In1)  "ui"
  Fbk/1 -> Sum/2  "Fbk"
  Saturation/1 -> Scope1/1, PI_Out (D)/1, Unit Delay1/1
  Merge1/1 -> Sum2/1, Unit Delay/1  "ui"
  Sum/1 -> Ki/1, Sum2/2  "Err"
  If Action Subsystem1/1(Out1) -> Merge1/1

== system Monorail_Auxiliary_Power_Unit/Second Stage/Pulse Generator/Current Loop/I PI Block/PI_MACRO (for Q) ==
  Ref : Inport
  Fbk : Inport  Port=2
  If Action Subsystem1 : Subsystem  TreatAsAtomicUnit=on
  If Action Subsystem3 : Subsystem  TreatAsAtomicUnit=on
  If1 : If  NumInputs=2  IfExpression=u1 == u2
  Ki : Gain  Gain=Ki_Iinv
  Kp : Gain  Gain=Kp_Iinv
  Merge1 : Merge
  Saturation : Saturate  UpperLimit=PI_inv_max  LowerLimit=PI_inv_min
  Scope : Scope
  Scope1 : Scope
  Sum : Sum  Inputs=|+-
  Sum1 : Sum  Inputs=|++
  Sum2 : Sum  Inputs=|++
  Unit Delay : UnitDelay  SampleTime=-1  HasFrameUpgradeWarning=on
  Unit Delay1 : UnitDelay  SampleTime=-1  HasFrameUpgradeWarning=on
  Unit Delay2 : UnitDelay  SampleTime=-1  HasFrameUpgradeWarning=on
  PI_Out (Q) : Outport
  wires:
  Unit Delay2/1 -> [V1]
  Unit Delay1/1 -> [Out]
  Saturation/1 -> PI_Out (Q)/1, Unit Delay1/1, Scope1/1
  If Action Subsystem1/1(Out1) -> Merge1/1
  Sum/1 -> Sum2/2, Ki/1  "Err"
  Merge1/1 -> Unit Delay/1, Sum2/1  "ui"
  Fbk/1 -> Sum/2  "Fbk"
  Sum1/1 -> If Action Subsystem1/1(In1)  "ui"
  [V1] -> If1/2
  Unit Delay/1 -> Sum1/2, If Action Subsystem3/1(In1)  "i1"
  If1/1 -> If Action Subsystem1/Action
  [Out] -> If1/1
  Kp/1 -> Saturation/1, Unit Delay2/1, Scope/1
  Ki/1 -> Sum1/1  "Ki*Err"
  Ref/1 -> Sum/1  "Ref"
  If1/2 -> If Action Subsystem3/Action
  Sum2/1 -> Kp/1  "Err+ui"
  If Action Subsystem3/1(Out1) -> Merge1/2

== system Monorail_Auxiliary_Power_Unit/Second Stage/Pulse Generator/Pulse/SVGEN_DQ/Scaling Block ==
  In : Inport
  Constant : Constant
  Gain : Gain  Gain=1/2
  Sum : Sum  Inputs=|++
  Out : Outport
  wires:
  Sum/1 -> Gain/1
  Constant/1 -> Sum/2
  In/1 -> Sum/1
  Gain/1 -> Out/1

== system Monorail_Auxiliary_Power_Unit/Second Stage/Pulse Generator/Pulse/SVGEN_DQ/Sector Determination ==
  Temp : Inport
  Constant3 : Constant  Value=3
  Demux : Demux  Outputs=3
  If Action Subsystem : Subsystem  TreatAsAtomicUnit=on
  If Action Subsystem1 : Subsystem  TreatAsAtomicUnit=on
  If Action Subsystem2 : Subsystem  TreatAsAtomicUnit=on
  If Action Subsystem3 : Subsystem  TreatAsAtomicUnit=on
  If Action Subsystem4 : Subsystem  TreatAsAtomicUnit=on
  If Action Subsystem5 : Subsystem  TreatAsAtomicUnit=on
  If1 : If
  If2 : If
  If3 : If  IfExpression=u1 < 0
  Merge1 : Merge
  Merge2 : Merge
  Merge3 : Merge
  Sector : Outport
  wires:
  If2/1 -> If Action Subsystem2/Action
  If Action Subsystem2/1(Out1) -> Merge2/1
  Merge2/1 -> If Action Subsystem4/1(In1), If Action Subsystem5/1(In1)
  Merge1/1 -> If Action Subsystem3/1(In1), If Action Subsystem2/1(In1)
  If1/1 -> If Action Subsystem/Action
  If Action Subsystem3/1(Out1) -> Merge2/2
  If1/2 -> If Action Subsystem1/Action
  Constant3/1 -> If Action Subsystem/1(In1), If Action Subsystem1/1(In1)
  If Action Subsystem4/1(Out1) -> Merge3/1
  If Action Subsystem/1(Out1) -> Merge1/1
  If3/1 -> If Action Subsystem4/Action
  If3/2 -> If Action Subsystem5/Action
  If Action Subsystem5/1(Out1) -> Merge3/2
  If2/2 -> If Action Subsystem3/Action
  Merge3/1 -> Sector/1
  If Action Subsystem1/1(Out1) -> Merge1/2
  Demux/1 -> [tmp1]  "tmp1"
  Demux/3 -> [tmp3]  "tmp3"
  Demux/2 -> [tmp2]  "tmp2"
  Temp/1 -> Demux/1
  [tmp1] -> If3/1
  [tmp2] -> If1/1
  [tmp3] -> If2/1

== system Monorail_Auxiliary_Power_Unit/Second Stage/Pulse Generator/Pulse/SVGEN_DQ/Switching Time Calculation ==
  tmp : Inport
  Sector : Inport  Port=2
  If : If  IfExpression=u1==1 | u1==4  ElseIfExpressions=u1==2 | u1==5
  If Action Subsystem6 : Subsystem  TreatAsAtomicUnit=on
  If Action Subsystem7 : Subsystem  TreatAsAtomicUnit=on
  If Action Subsystem8 : Subsystem  TreatAsAtomicUnit=on
  Merge : Merge  Inputs=3
  Switching Time : Outport
  wires:
  If Action Subsystem6/1(Out1) -> Merge/1
  If Action Subsystem8/1(Out1) -> Merge/3
  If/3 -> If Action Subsystem8/Action
  If/2 -> If Action Subsystem7/Action
  If/1 -> If Action Subsystem6/Action
  tmp/1 -> If Action Subsystem6/1(In1), If Action Subsystem7/1(In1), If Action Subsystem8/1(In1)
  If Action Subsystem7/1(Out1) -> Merge/2
  Sector/1 -> If/1
  Merge/1 -> Switching Time/1

== system Monorail_Auxiliary_Power_Unit/Second Stage/Pulse Generator/Pulse/SVGEN_DQ/Temp calculation ==
  Alpha : Inport
  Beta : Inport  Port=2
  Add : Sum
  Add1 : Sum  Inputs=+-
  Gain : Gain  Gain=1/2
  Gain1 : Gain  Gain=sqrt(3)/2
  Mux2 : Mux  Inputs=3
  Scope1 : Scope  NumInputPorts=3
  Temp : Outport
  wires:
  Mux2/1 -> Temp/1
  Beta/1 -> Scope1/1, Mux2/1, Add1/2, Gain/1  "temp1"
  Add/1 -> Mux2/2, Scope1/2, Add1/1  "temp2"
  Add1/1 -> Mux2/3, Scope1/3  "temp3"
  Gain1/1 -> Add/1
  Gain/1 -> Add/2
  Alpha/1 -> Gain1/1

== system Monorail_Auxiliary_Power_Unit/Second Stage/Pulse Generator/Voltage Loop/V PI Block/PI_MACRO (for 0) ==
  Ref : Inport
  Fbk : Inport  Port=2
  If Action Subsystem1 : Subsystem  TreatAsAtomicUnit=on
  If Action Subsystem3 : Subsystem  TreatAsAtomicUnit=on
  If1 : If  NumInputs=2  IfExpression=u1 == u2
  Ki : Gain  Gain=Ki_inv
  Kp : Gain  Gain=Kp_inv
  Merge1 : Merge
  Saturation : Saturate  UpperLimit=PI_inv_max  LowerLimit=PI_inv_min
  Scope : Scope
  Scope1 : Scope
  Sum : Sum  Inputs=|+-
  Sum1 : Sum  Inputs=|++
  Sum2 : Sum  Inputs=|++
  Unit Delay : UnitDelay  SampleTime=-1  HasFrameUpgradeWarning=on
  Unit Delay1 : UnitDelay  SampleTime=-1  HasFrameUpgradeWarning=on
  Unit Delay2 : UnitDelay  SampleTime=-1  HasFrameUpgradeWarning=on
  PI_Out (0) : Outport
  wires:
  Unit Delay2/1 -> [V1]
  Unit Delay1/1 -> [Out]
  Saturation/1 -> Scope1/1, PI_Out (0)/1, Unit Delay1/1
  If Action Subsystem1/1(Out1) -> Merge1/1
  Sum/1 -> Sum2/2, Ki/1  "Err"
  Merge1/1 -> Unit Delay/1, Sum2/1  "ui"
  Fbk/1 -> Sum/2  "Fbk"
  Sum1/1 -> If Action Subsystem1/1(In1)  "ui"
  [V1] -> If1/2
  Unit Delay/1 -> Sum1/2, If Action Subsystem3/1(In1)  "i1"
  If1/1 -> If Action Subsystem1/Action
  [Out] -> If1/1
  Kp/1 -> Scope/1, Saturation/1, Unit Delay2/1
  Ki/1 -> Sum1/1  "Ki*Err"
  Ref/1 -> Sum/1  "Ref"
  If1/2 -> If Action Subsystem3/Action
  Sum2/1 -> Kp/1  "Err+ui"
  If Action Subsystem3/1(Out1) -> Merge1/2

== system Monorail_Auxiliary_Power_Unit/Second Stage/Pulse Generator/Voltage Loop/V PI Block/PI_MACRO (for D) ==
  Ref : Inport
  Fbk : Inport  Port=2
  If Action Subsystem1 : Subsystem  TreatAsAtomicUnit=on
  If Action Subsystem3 : Subsystem  TreatAsAtomicUnit=on
  If1 : If  NumInputs=2  IfExpression=u1 == u2
  Ki : Gain  Gain=Ki_inv
  Kp : Gain  Gain=Kp_inv
  Merge1 : Merge
  Saturation : Saturate  UpperLimit=PI_inv_max  LowerLimit=PI_inv_min
  Scope : Scope
  Scope1 : Scope
  Sum : Sum  Inputs=|+-
  Sum1 : Sum  Inputs=|++
  Sum2 : Sum  Inputs=|++
  Unit Delay : UnitDelay  SampleTime=-1  HasFrameUpgradeWarning=on
  Unit Delay1 : UnitDelay  SampleTime=-1  HasFrameUpgradeWarning=on
  Unit Delay2 : UnitDelay  SampleTime=-1  HasFrameUpgradeWarning=on
  PI_Out (D) : Outport
  wires:
  If Action Subsystem1/1(Out1) -> Merge1/1
  Sum/1 -> Sum2/2, Ki/1  "Err"
  Merge1/1 -> Unit Delay/1, Sum2/1  "ui"
  Saturation/1 -> Unit Delay1/1, PI_Out (D)/1, Scope1/1
  Fbk/1 -> Sum/2  "Fbk"
  Sum1/1 -> If Action Subsystem1/1(In1)  "ui"
  [V1] -> If1/2
  Unit Delay/1 -> Sum1/2, If Action Subsystem3/1(In1)  "i1"
  If1/1 -> If Action Subsystem1/Action
  [Out] -> If1/1
  Kp/1 -> Saturation/1, Scope/1, Unit Delay2/1
  Ki/1 -> Sum1/1  "Ki*Err"
  Ref/1 -> Sum/1  "Ref"
  If1/2 -> If Action Subsystem3/Action
  Sum2/1 -> Kp/1  "Err+ui"
  If Action Subsystem3/1(Out1) -> Merge1/2
  Unit Delay1/1 -> [Out]
  Unit Delay2/1 -> [V1]

== system Monorail_Auxiliary_Power_Unit/Second Stage/Pulse Generator/Voltage Loop/V PI Block/PI_MACRO (for Q) ==
  Ref : Inport
  Fbk : Inport  Port=2
  If Action Subsystem1 : Subsystem  TreatAsAtomicUnit=on
  If Action Subsystem3 : Subsystem  TreatAsAtomicUnit=on
  If1 : If  NumInputs=2  IfExpression=u1 == u2
  Ki : Gain  Gain=Ki_inv
  Kp : Gain  Gain=Kp_inv
  Merge1 : Merge
  Saturation : Saturate  UpperLimit=PI_inv_max  LowerLimit=PI_inv_min
  Scope : Scope
  Scope1 : Scope
  Sum : Sum  Inputs=|+-
  Sum1 : Sum  Inputs=|++
  Sum2 : Sum  Inputs=|++
  Unit Delay : UnitDelay  SampleTime=-1  HasFrameUpgradeWarning=on
  Unit Delay1 : UnitDelay  SampleTime=-1  HasFrameUpgradeWarning=on
  Unit Delay2 : UnitDelay  SampleTime=-1  HasFrameUpgradeWarning=on
  PI_Out (Q) : Outport
  wires:
  If Action Subsystem3/1(Out1) -> Merge1/2
  Sum2/1 -> Kp/1  "Err+ui"
  If1/2 -> If Action Subsystem3/Action
  Ref/1 -> Sum/1  "Ref"
  Ki/1 -> Sum1/1  "Ki*Err"
  Kp/1 -> Scope/1, Unit Delay2/1, Saturation/1
  [Out] -> If1/1
  If1/1 -> If Action Subsystem1/Action
  Unit Delay/1 -> If Action Subsystem3/1(In1), Sum1/2  "i1"
  [V1] -> If1/2
  Sum1/1 -> If Action Subsystem1/1(In1)  "ui"
  Fbk/1 -> Sum/2  "Fbk"
  Merge1/1 -> Sum2/1, Unit Delay/1  "ui"
  Sum/1 -> Ki/1, Sum2/2  "Err"
  If Action Subsystem1/1(Out1) -> Merge1/1
  Saturation/1 -> Scope1/1, Unit Delay1/1, PI_Out (Q)/1
  Unit Delay1/1 -> [Out]
  Unit Delay2/1 -> [V1]

== system Monorail_Auxiliary_Power_Unit/First Stage/PSFB Pulse Generator/Voltage Loop/Close Loop/Feedback/Error Signal Generator ==
  V dc : Inport
  V bat : Inport  Port=2
  Fbk Sel : Inport  Port=3
  Gain : Gain  Gain=Scale_factor_High
  Gain1 : Gain  Gain=Scale_factor_High
  Gain2 : Gain  Gain=Scale_factor_Low
  Gain3 : Gain  Gain=Scale_factor_Low
  Ramp : simulink/Sources/Ramp  slope=V_dc_ref/t_softstart  start=0  InitialOutput=0
  Ramp1 : simulink/Sources/Ramp  slope=V_bat_ref/t_softstart  start=0  InitialOutput=0
  Saturation1 : Saturate  UpperLimit=V_dc_ref  LowerLimit=V_dc_init  ZeroCross=off
  Saturation3 : Saturate  UpperLimit=V_bat_ref  LowerLimit=V_bat_init  ZeroCross=off
  Sum : Sum  Inputs=|+-
  Sum1 : Sum  Inputs=|+-
  Switch : Switch  Criteria=u2 > Threshold  Threshold=1/2
  Error Signal : Outport
  wires:
  Sum/1 -> Switch/1
  Saturation3/1 -> Gain2/1
  Saturation1/1 -> Gain/1
  Gain2/1 -> Sum1/1
  Ramp/1 -> Saturation1/1
  Gain/1 -> Sum/1
  Gain1/1 -> Sum/2
  Gain3/1 -> Sum1/2
  Ramp1/1 -> Saturation3/1
  Sum1/1 -> Switch/3
  V dc/1 -> Gain1/1
  Fbk Sel/1 -> Switch/2
  V bat/1 -> Gain3/1
  Switch/1 -> Error Signal/1

== system Monorail_Auxiliary_Power_Unit/First Stage/PSFB Pulse Generator/Voltage Loop/Close Loop/Feedback/PI Controller ==
  PI In : Inport
  Gain : Gain  Gain=Ki_psfb
  Gain1 : Gain  Gain=Kp_psfb
  Integrator : Integrator
  Saturation2 : Saturate  UpperLimit=PI_max  LowerLimit=PI_min  ZeroCross=off
  Sum : Sum
  Sum1 : Sum  Inputs=|++
  PI Out : Outport
  wires:
  PI In/1 -> Sum/1, Gain1/1
  Saturation2/1 -> PI Out/1
  Sum/1 -> Integrator/1, Gain/1
  Integrator/1 -> Sum/2
  Gain1/1 -> Sum1/1
  Gain/1 -> Sum1/2
  Sum1/1 -> Saturation2/1

== system Monorail_Auxiliary_Power_Unit/Second Stage/Pulse Generator/Current Loop/I PI Block/PI_MACRO (for 0)/If Action Subsystem1 ==
  In1 : Inport
  Action Port : ActionPort  ActionPortLabel=if(u1 == u2)
  Out1 : Outport
  wires:
  In1/1 -> Out1/1

== system Monorail_Auxiliary_Power_Unit/Second Stage/Pulse Generator/Current Loop/I PI Block/PI_MACRO (for 0)/If Action Subsystem3 ==
  In1 : Inport
  Action Port : ActionPort  ActionPortLabel=else
  Out1 : Outport
  wires:
  In1/1 -> Out1/1

== system Monorail_Auxiliary_Power_Unit/Second Stage/Pulse Generator/Current Loop/I PI Block/PI_MACRO (for D)/If Action Subsystem1 ==
  In1 : Inport
  Action Port : ActionPort  ActionPortLabel=if(u1 == u2)
  Out1 : Outport
  wires:
  In1/1 -> Out1/1

== system Monorail_Auxiliary_Power_Unit/Second Stage/Pulse Generator/Current Loop/I PI Block/PI_MACRO (for D)/If Action Subsystem3 ==
  In1 : Inport
  Action Port : ActionPort  ActionPortLabel=else
  Out1 : Outport
  wires:
  In1/1 -> Out1/1

== system Monorail_Auxiliary_Power_Unit/Second Stage/Pulse Generator/Current Loop/I PI Block/PI_MACRO (for Q)/If Action Subsystem1 ==
  In1 : Inport
  Action Port : ActionPort  ActionPortLabel=if(u1 == u2)
  Out1 : Outport
  wires:
  In1/1 -> Out1/1

== system Monorail_Auxiliary_Power_Unit/Second Stage/Pulse Generator/Current Loop/I PI Block/PI_MACRO (for Q)/If Action Subsystem3 ==
  In1 : Inport
  Action Port : ActionPort  ActionPortLabel=else
  Out1 : Outport
  wires:
  In1/1 -> Out1/1

== system Monorail_Auxiliary_Power_Unit/Second Stage/Pulse Generator/Pulse/SVGEN_DQ/Sector Determination/If Action Subsystem ==
  In1 : Inport
  Action Port : ActionPort  ActionPortLabel=if(u1 > 0)
  Constant : Constant
  Subtract : Sum  Inputs=+-
  Out1 : Outport
  wires:
  In1/1 -> Subtract/1
  Constant/1 -> Subtract/2
  Subtract/1 -> Out1/1

== system Monorail_Auxiliary_Power_Unit/Second Stage/Pulse Generator/Pulse/SVGEN_DQ/Sector Determination/If Action Subsystem1 ==
  In1 : Inport
  Action Port : ActionPort  ActionPortLabel=else
  Out1 : Outport
  wires:
  In1/1 -> Out1/1

== system Monorail_Auxiliary_Power_Unit/Second Stage/Pulse Generator/Pulse/SVGEN_DQ/Sector Determination/If Action Subsystem2 ==
  In1 : Inport
  Action Port : ActionPort  ActionPortLabel=if(u1 > 0)
  Constant : Constant
  Subtract : Sum  Inputs=+-
  Out1 : Outport
  wires:
  Subtract/1 -> Out1/1
  Constant/1 -> Subtract/2
  In1/1 -> Subtract/1

== system Monorail_Auxiliary_Power_Unit/Second Stage/Pulse Generator/Pulse/SVGEN_DQ/Sector Determination/If Action Subsystem3 ==
  In1 : Inport
  Action Port : ActionPort  ActionPortLabel=else
  Out1 : Outport
  wires:
  In1/1 -> Out1/1

== system Monorail_Auxiliary_Power_Unit/Second Stage/Pulse Generator/Pulse/SVGEN_DQ/Sector Determination/If Action Subsystem4 ==
  In1 : Inport
  Action Port : ActionPort  ActionPortLabel=if(u1 < 0)
  Constant : Constant  Value=7
  Subtract : Sum  Inputs=-+
  Out1 : Outport
  wires:
  In1/1 -> Subtract/1
  Constant/1 -> Subtract/2
  Subtract/1 -> Out1/1

== system Monorail_Auxiliary_Power_Unit/Second Stage/Pulse Generator/Pulse/SVGEN_DQ/Sector Determination/If Action Subsystem5 ==
  In1 : Inport
  Action Port : ActionPort  ActionPortLabel=else
  Out1 : Outport
  wires:
  In1/1 -> Out1/1

== system Monorail_Auxiliary_Power_Unit/Second Stage/Pulse Generator/Pulse/SVGEN_DQ/Switching Time Calculation/If Action Subsystem6 ==
  In1 : Inport
  Action Port : ActionPort  ActionPortLabel=if(u1==1 | u1==4)
  Add : Sum  Inputs=+-
  Demux : Demux  Outputs=3
  Gain : Gain  Gain=-1
  Mux : Mux  Inputs=3
  Out1 : Outport
  wires:
  In1/1 -> Demux/1
  Demux/2 -> Gain/1, Mux/1
  Demux/1 -> Add/1
  Demux/3 -> Add/2
  Add/1 -> Mux/2
  Gain/1 -> Mux/3
  Mux/1 -> Out1/1
